simulink model "agws"  (R2016a)
settings: Solver=FixedStepDiscrete  StartTime=0.0  StopTime=50  FixedStep=0.1  RelTol=1e-3
values from neighbouring files (symbols this model uses):
  M1_BeMo_d = zeros(7,M1_n_mode)    [AcO_Ctrl_headless_cfg.m]    (also in agws_cfg.m = 1e-6*bsxfun(@times,randn(7,M1_n_mode),scale); agws_fastTT_cfg.m = 1e-6*bsxfun(@times,randn(7,M1_n_mode),scale))
  M1_RiBo_d = zeros(7,6)    [AcO_Ctrl_headless_cfg.m]    (also in agws_cfg.m = [M1_Txyz0 M1_Rxyz0]; agws_fastTT_cfg.m = [M1_Txyz0 M1_Rxyz0])
  M2_RiBo_d = zeros(7,6)    [AcO_Ctrl_headless_cfg.m]    (also in agws_cfg.m = [M2_Txyz0 M2_Rxyz0]; agws_fastTT_cfg.m = [M2_Txyz0 M2_Rxyz0])
undefined symbols (not defined in the file or in its folder): R
libraries: CEO x5
settings Model: Creator=rconan  LastModifiedBy=rconan
settings DataIOCC: LimitDataPoints=on  SaveFormat=Array
settings HardwareCC: ProdBitPerPointer=32  ProdLargestAtomicFloat=None  ProdIntDivRoundTo=Undefined  ProdEndianess=Unspecified  ProdWordSize=32  ProdHWDeviceType=32-bit Generic
settings ModelReferenceCC: PropagateSignalLabelsOutOfModel=off
settings ConfigComp: CovModelRefEnable=Off

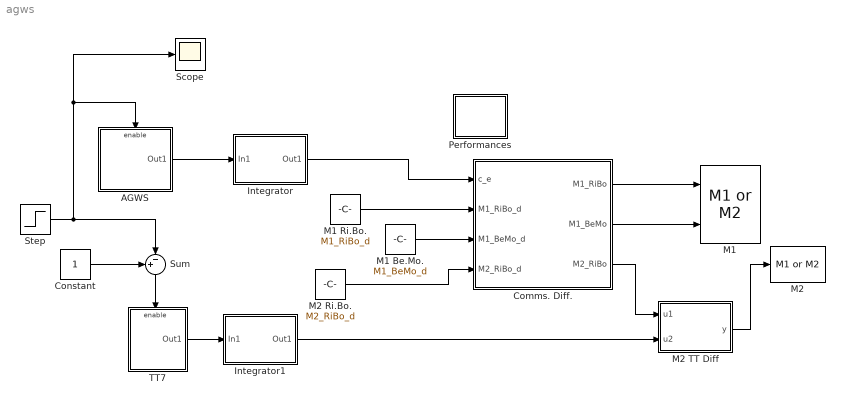
== system agws ==
  AGWS : Subsystem
  Comms. Diff. : MATLAB Function  TreatAsAtomicUnit=on
  Constant : Constant
  Integrator : Subsystem
  Integrator1 : Subsystem
  M1 : CEO/M1 or M2  mirror=M1  TxyzRxyz=on  mode_coefs=on  n_mode=42  sampleTime=[-1,0]
  M1 Be.Mo. : Constant  Value=M1_BeMo_d
  M1 Ri.Bo. : Constant  Value=M1_RiBo_d
  M2 : CEO/M1 or M2  mirror=M2  TxyzRxyz=on  mode_coefs=off  n_mode=66  sampleTime=[-1,0]
  M2 Ri.Bo. : Constant  Value=M2_RiBo_d
  M2 TT Diff : MATLAB Function  TreatAsAtomicUnit=on
  Performances : Subsystem
  Scope : Scope
  Step : Step  Time=0  SampleTime=1
  Sum : Sum  Inputs=+-|
  TT7 : Subsystem
  wires:
  M1 Ri.Bo./1 -> Comms. Diff./2(M1_RiBo_d)
  Comms. Diff./1(M1_RiBo) -> M1/1
  Comms. Diff./2(M1_BeMo) -> M1/2
  M2 Ri.Bo./1 -> Comms. Diff./4(M2_RiBo_d)
  M1 Be.Mo./1 -> Comms. Diff./3(M1_BeMo_d)
  Integrator/1(Out1) -> Comms. Diff./1(c_e)
  Integrator1/1(Out1) -> M2 TT Diff/2(u2)
  M2 TT Diff/1(y) -> M2/1
  Comms. Diff./3(M2_RiBo) -> M2 TT Diff/1(u1)
  TT7/1(Out1) -> Integrator1/1(In1)
  Sum/1 -> TT7/Enable
  Step/1 -> AGWS/Enable, Scope/1, Sum/2
  Constant/1 -> Sum/1
  AGWS/1(Out1) -> Integrator/1(In1)

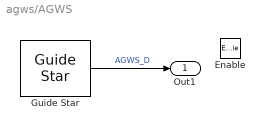
== system agws/AGWS ==
  Enable : EnablePort
  Guide Star : CEO/Guide Star  zenith=gs_zen  azimuth=gs_azi  photometry=R - 0.640  magnitude=0  rays_origin=[0,0,25]  rays_box_size=25.5  rays_box_sampling=16  sensor=GeometricShackHartmann  fwhm=[]  sampleTime=[1,0]  n_lenslet=30  d=26/30  n_cam=128  px_scale=NaN  intensity_threshold=0.2  a=1  b=1  wfe_rms=off  segment_wfe_rms=off  piston=off  segment_piston=off  tiptilt=off  segment_tiptilt=off  ee80=off  sens=off  calibration_file='AGWS_Calibration'  coms=gs_calib  coms_size=gs_calib_size  svd_truncation=6
  Out1 : Outport
  wires:
  Guide Star/1 -> Out1/1  "AGWS_D"

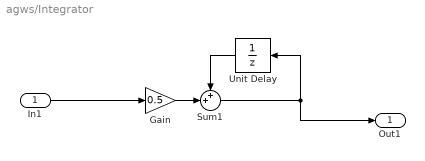
== system agws/Integrator ==
  In1 : Inport
  Gain : Gain  Gain=0.5
  Sum1 : Sum  Inputs=++|
  Unit Delay : UnitDelay  SampleTime=-1
  Out1 : Outport
  wires:
  In1/1 -> Gain/1
  Gain/1 -> Sum1/2
  Unit Delay/1 -> Sum1/1
  Sum1/1 -> Out1/1, Unit Delay/1

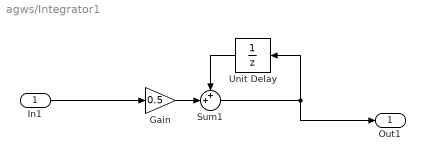
== system agws/Integrator1 ==
  In1 : Inport
  Gain : Gain  Gain=0.5
  Sum1 : Sum  Inputs=++|
  Unit Delay : UnitDelay  SampleTime=-1
  Out1 : Outport
  wires:
  In1/1 -> Gain/1
  Gain/1 -> Sum1/2
  Unit Delay/1 -> Sum1/1
  Sum1/1 -> Out1/1, Unit Delay/1

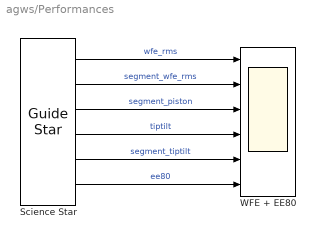
== system agws/Performances ==
  Science Star : CEO/Guide Star  zenith=0  azimuth=0  photometry=R - 0.640  magnitude=0  rays_origin=[0,0,25]  rays_box_size=25.5  rays_box_sampling=256  sensor=Imaging  fwhm=[]  sampleTime=[1,0]  n_lenslet=1  d=26  n_cam=128  px_scale=0.00127  intensity_threshold=0.5  a=2  b=1  wfe_rms=on  segment_wfe_rms=on  piston=off  segment_piston=on  tiptilt=on  segment_tiptilt=on  ee80=on  sens=off  calibration_file=[]  coms=[]  coms_size=14  svd_truncation=0
  WFE + EE80 : Scope  NumInputPorts=6
  wires:
  Science Star/3 -> WFE + EE80/3  "segment_piston"
  Science Star/5 -> WFE + EE80/5  "segment_tiptilt"
  Science Star/4 -> WFE + EE80/4  "tiptilt"
  Science Star/2 -> WFE + EE80/2  "segment_wfe_rms"
  Science Star/1 -> WFE + EE80/1  "wfe_rms"
  Science Star/6 -> WFE + EE80/6  "ee80"

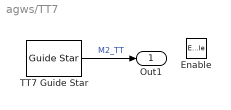
== system agws/TT7 ==
  Enable : EnablePort
  TT7 Guide Star : CEO/Guide Star  zenith=0  azimuth=0  photometry=R - 0.640  magnitude=0  rays_origin=[0,0,25]  rays_box_size=25.5  rays_box_sampling=8  sensor=TT7  fwhm=[]  sampleTime=[1,0]  n_lenslet=30  d=1  n_cam=128  px_scale=0.066  intensity_threshold=0.5  a=1  b=1  wfe_rms=off  segment_wfe_rms=off  piston=off  segment_piston=off  tiptilt=off  segment_tiptilt=off  ee80=off  sens=off  calibration_file=[]  coms=struct('M2_TT',struct('mirror','M2','mode','segment tip-tilt','stroke',1e-6))  coms_size=14  svd_truncation=0
  Out1 : Outport
  wires:
  TT7 Guide Star/1 -> Out1/1  "M2_TT"

== matlab function agws/M2 TT Diff ==
  data: u1 input; y output; u2 input
function y = M2TTrm(u1,u2)
%#codegen

y = u1;
y(:,4:5) = u1(:,4:5) - reshape(u2,2,7)';

== matlab function agws/Comms. Diff. ==
  data: c_e input; M1_RiBo output; M1_RiBo_d input; M1_BeMo output; M1_BeMo_d input; M2_RiBo output; M2_RiBo_d input
function [M1_RiBo,M1_BeMo,M2_RiBo]= diff(c_e,M1_RiBo_d,M1_BeMo_d,M2_RiBo_d)
%#codegen

M1_Txyz = zeros(1,21);
M1_Rxyz = zeros(1,21);
M2_Rxyz = zeros(1,21);

M1_Rxyz(1:20) = c_e(1:20);
M2_Rxyz(1:20) = c_e(21:40);
M1_Txyz(1:20) = c_e(41:60);
M2_Txyz       = c_e(61:81);

M1_TR = [ reshape(M1_Txyz,3,7) ; reshape(M1_Rxyz,3,7) ];
%M1_TR = reshape( M1_TR, 1 , 42);

M2_TR = [ reshape(M2_Txyz,3,7) ; reshape(M2_Rxyz,3,7) ];
%M2_TR = reshape( M2_TR, 1 , 42);

M1_RiBo = M1_RiBo_d - M1_TR';
M2_RiBo = M2_RiBo_d - M2_TR';

M1_BeMo = M1_BeMo_d - reshape(c_e(82:end),[],7)';
